simulink model "model_test"  (R2017a)
settings: Solver=VariableStepAuto  StartTime=0.0  StopTime=10.0  RelTol=1e-3
values from neighbouring files (symbols this model uses):
  g = 9.81    [model_test.m]
  K = place(A,B,P)    [model_test.m]
  l = 0.8048    [model_test.m]
  m = 1    [model_test.m]
settings Model: Creator=Merc  LastModifiedBy=Merc

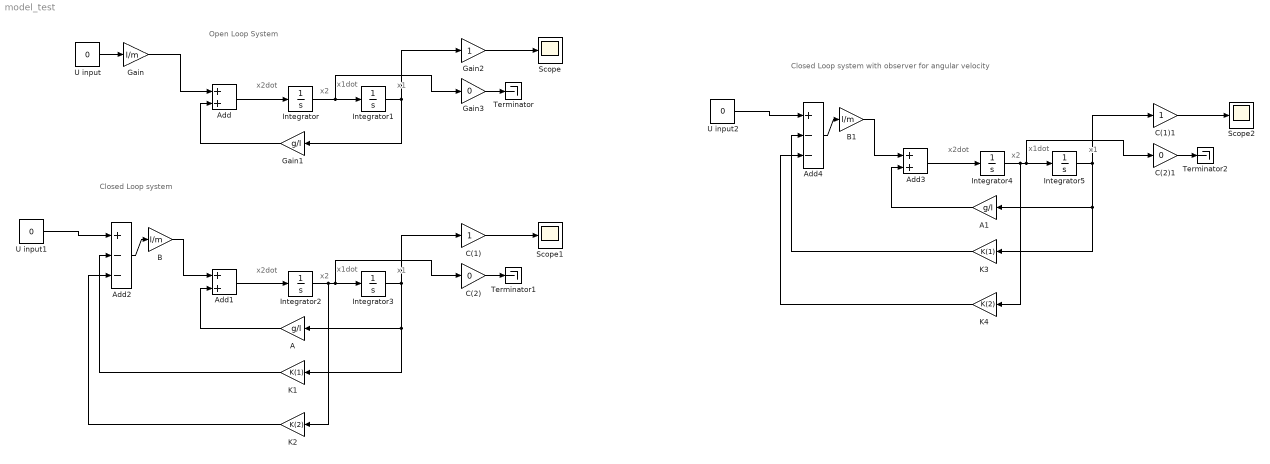
== system model_test ==
  note: Closed Loop system
  note: Open Loop System
  note: x1
  note: x1dot
  note: x2
  note: x2dot
  note: x1dot
  note: x2dot
  note: x2
  note: x1
  note: x1dot
  note: x2dot
  note: x2
  note: x1
  note: Closed Loop system with observer for angular velocity
  A : Gain  Gain=g/l
  A1 : Gain  Gain=g/l
  Add : Sum
  Add1 : Sum
  Add2 : Sum  Inputs=+--
  Add3 : Sum
  Add4 : Sum  Inputs=+--
  B : Gain  Gain=l/m
  B1 : Gain  Gain=l/m
  C(1) : Gain
  C(1)1 : Gain
  C(2) : Gain  Gain=0
  C(2)1 : Gain  Gain=0
  Gain : Gain  Gain=l/m
  Gain1 : Gain  Gain=g/l
  Gain2 : Gain
  Gain3 : Gain  Gain=0
  Integrator{,1..5} (6 alike) : Integrator  InitialCondition=1
  K1 : Gain  Gain=K(1)
  K2 : Gain  Gain=K(2)
  K3 : Gain  Gain=K(1)
  K4 : Gain  Gain=K(2)
  Scope : Scope
  Scope1 : Scope
  Scope2 : Scope
  Terminator : Terminator
  Terminator1 : Terminator
  Terminator2 : Terminator
  U input : Constant  Value=0
  U input1 : Constant  Value=0
  U input2 : Constant  Value=0
  wires:
  U input/1 -> Gain/1
  Gain/1 -> Add/1
  Add/1 -> Integrator/1
  Integrator/1 -> Gain3/1, Integrator1/1
  Integrator1/1 -> Gain1/1, Gain2/1
  Gain1/1 -> Add/2
  Gain3/1 -> Terminator/1
  Gain2/1 -> Scope/1
  Integrator2/1 -> K2/1, C(2)/1, Integrator3/1
  B/1 -> Add1/1
  C(1)/1 -> Scope1/1
  A/1 -> Add1/2
  C(2)/1 -> Terminator1/1
  Add1/1 -> Integrator2/1
  Integrator3/1 -> K1/1, A/1, C(1)/1
  Add2/1 -> B/1
  U input1/1 -> Add2/1
  K1/1 -> Add2/2
  K2/1 -> Add2/3
  B1/1 -> Add3/1
  Integrator5/1 -> K3/1, A1/1, C(1)1/1
  Add3/1 -> Integrator4/1
  Add4/1 -> B1/1
  C(1)1/1 -> Scope2/1
  C(2)1/1 -> Terminator2/1
  U input2/1 -> Add4/1
  K4/1 -> Add4/3
  Integrator4/1 -> K4/1, C(2)1/1, Integrator5/1
  K3/1 -> Add4/2
  A1/1 -> Add3/2
